simulink model "boost_inverter_control"  (R2018a)
settings: Solver=FixedStepAuto  StartTime=0.0  StopTime=0.5  FixedStep=1e-5  RelTol=1e-3  EnableMultiTasking=on
undefined symbols (not defined in the file): a, C, ki, kp, L, R, Wg
libraries: powerlib_meascontrol x4, simulink x1
settings Model: Creator=PC  LastModifiedBy=yassine
settings OptimizationCC: LifeSpan=inf
settings DebuggingCC: SFUnexpectedBacktrackingDiag=warning  SFNoUnconditionalDefaultTransitionDiag=warning
settings CodeAppCC: StateflowObjectComments=on
settings GRTTargetCC: TargetLangStandard=C89/C90 (ANSI)
settings ConfigComp: CovMetricSettings=dw  CovSaveCumulativeToWorkspaceVar=on  CovSaveSingleToWorkspaceVar=on  CovExternalEMLEnable=off

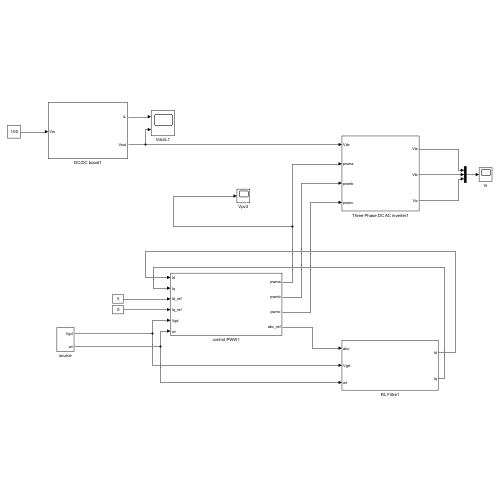
[thumbnail: Simulink's stored preview of the top-level diagram]
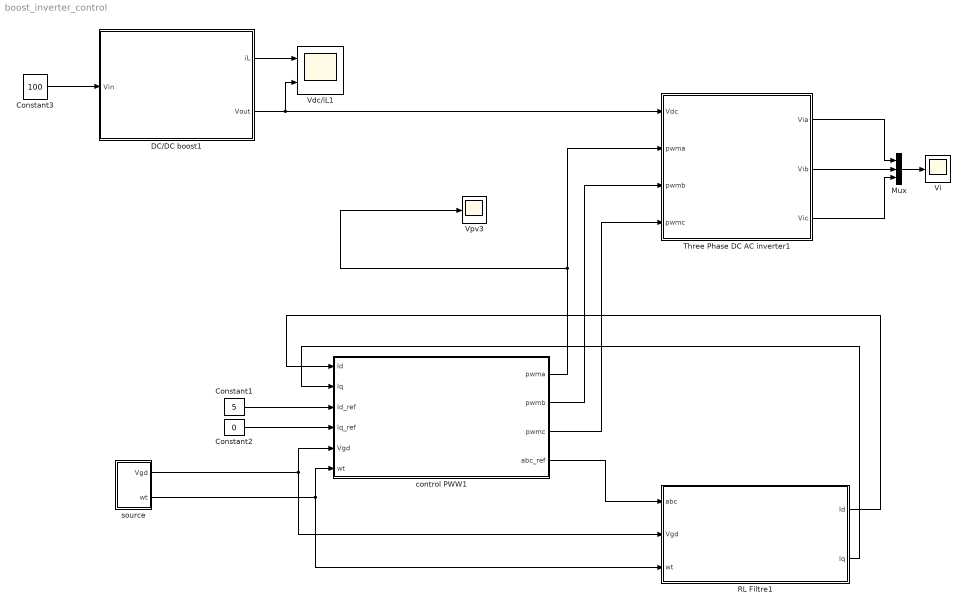
== system boost_inverter_control ==
  Constant1 : Constant  Value=5
  Constant2 : Constant  Value=0
  Constant3 : Constant  Value=100
  DC/DC boost1 : Subsystem  InitFcn=|
      | dv=0.5;
      | di=0.1;
      | F=20e3;
      | T=1/F;
      | Vs=230;
      | Vab=sqrt(3)*Vs;
      | Vdc=2*sqrt(2)*Vab/sqrt(3);
      | Vpv=100;
      | a=1-Vpv/Vdc;
      | Pn=200*5;
      | R=Vdc*Vdc/Pn;
      | L=0.5*Vpv*a*T/di;
      | C=0.5*Vdc*a*T/(dv*R);
  Mux : Mux  Inputs=3
  RL Filtre1 : Subsystem  InitFcn=|
      | fs=5000;
      | fe=50;
      | Wg=2*pi*fs;
      | Ig=2*Pn/(3*230*sqrt(2));
      | dIg=0.05*Ig;
      | L_=230*sqrt(3)/(6*sqrt(2)*fs*dIg);
      | r=0.01;
  Three Phase DC AC inverter1 : Subsystem
  Vdc/iL1 : Scope  NumInputPorts=2
  Vi : Scope
  Vpv3 : Scope
  control PWW1 : Subsystem  InitFcn=|
      | fs=5000;
      | fe=50;
      | Wg=2*pi*fe;
      | Ig=2*Pn/(3*230*sqrt(2));
      | dIg=0.05*Ig;
      | L=230*sqrt(3)/(6*sqrt(2)*fs*dIg);
      | Id_=5;
      | Iq_=0;
      | R=0.01;
      | tr=10e-5;
      | Te=tr/3;
      | ki=R/Te;
      | kp=L/Te;
  source : Subsystem
  wires:
  RL Filtre1/1(Id) -> control PWW1/1(Id)
  RL Filtre1/2(Iq) -> control PWW1/2(Iq)
  source/1(Vgd) -> control PWW1/5(Vgd), RL Filtre1/2(Vgd)
  Constant2/1 -> control PWW1/4(Iq_ref)
  Constant1/1 -> control PWW1/3(Id_ref)
  control PWW1/3(pwmc) -> Three Phase DC AC inverter1/4(pwmc)
  control PWW1/2(pwmb) -> Three Phase DC AC inverter1/3(pwmb)
  control PWW1/1(pwma) -> Three Phase DC AC inverter1/2(pwma), Vpv3/1
  DC/DC boost1/1(iL) -> Vdc/iL1/1
  Constant3/1 -> DC/DC boost1/1(Vin)
  Three Phase DC AC inverter1/1(Via) -> Mux/1
  Three Phase DC AC inverter1/2(Vib) -> Mux/2
  DC/DC boost1/2(Vout) -> Three Phase DC AC inverter1/1(Vdc), Vdc/iL1/2
  source/2(wt) -> control PWW1/6(wt), RL Filtre1/3(wt)
  control PWW1/4(abc_ref) -> RL Filtre1/1(abc)
  Mux/1 -> Vi/1
  Three Phase DC AC inverter1/3(Vic) -> Mux/3

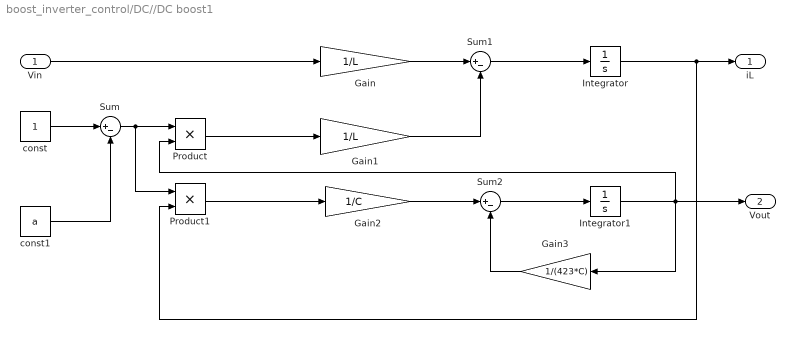
== system boost_inverter_control/DC//DC boost1 ==
  Vin : Inport
  Gain : Gain  Gain=1/L
  Gain1 : Gain  Gain=1/L
  Gain2 : Gain  Gain=1/C
  Gain3 : Gain  Gain=1/(423*C)
  Integrator : Integrator
  Integrator1 : Integrator
  Product : Product
  Product1 : Product
  Sum : Sum  Inputs=|+-
  Sum1 : Sum  Inputs=|+-
  Sum2 : Sum  Inputs=|+-
  const : Constant
  const1 : Constant  Value=a
  iL : Outport
  Vout : Outport  Port=2
  wires:
  Gain3/1 -> Sum2/2
  Integrator1/1 -> Vout/1, Product/2, Gain3/1
  Sum2/1 -> Integrator1/1
  Integrator/1 -> iL/1, Product1/2
  Vin/1 -> Gain/1
  const/1 -> Sum/1
  Product1/1 -> Gain2/1
  Product/1 -> Gain1/1
  Sum1/1 -> Integrator/1
  Gain1/1 -> Sum1/2
  Sum/1 -> Product/1, Product1/1
  Gain2/1 -> Sum2/1
  Gain/1 -> Sum1/1
  const1/1 -> Sum/2

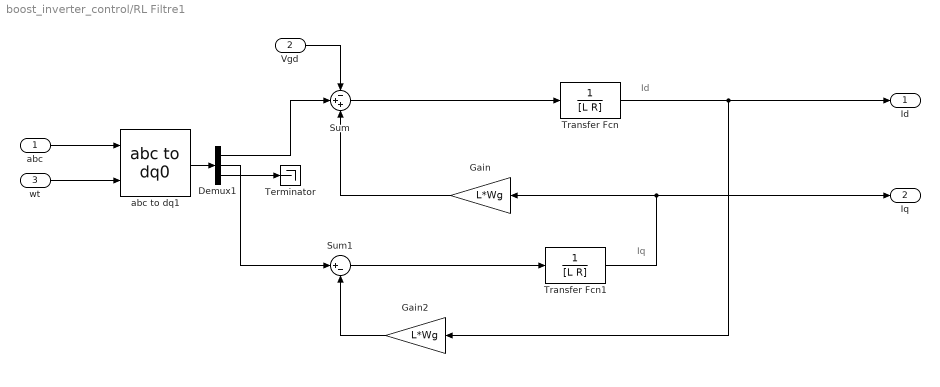
== system boost_inverter_control/RL Filtre1 ==
  note: Id
  note: Iq
  abc : Inport
  Vgd : Inport  Port=2
  wt : Inport  Port=3
  Demux1 : Demux  Outputs=3
  Gain : Gain  Gain=L*Wg
  Gain2 : Gain  Gain=L*Wg
  Sum : Sum  Inputs=-++
  Sum1 : Sum  Inputs=|+-
  Terminator : Terminator
  Transfer Fcn : TransferFcn  Denominator=[L R]
  Transfer Fcn1 : TransferFcn  Denominator=[L R]
  abc to dq1 : powerlib_meascontrol/Transformations/abc to dq0  Alignment=90 degrees behind phase A axis
  Id : Outport
  Iq : Outport  Port=2
  wires:
  Transfer Fcn/1 -> Gain2/1, Id/1
  Transfer Fcn1/1 -> Gain/1, Iq/1
  Demux1/1 -> Sum/2
  Demux1/2 -> Sum1/1
  abc to dq1/1 -> Demux1/1
  Demux1/3 -> Terminator/1
  abc/1 -> abc to dq1/1
  wt/1 -> abc to dq1/2
  Sum/1 -> Transfer Fcn/1
  Sum1/1 -> Transfer Fcn1/1
  Vgd/1 -> Sum/1
  Gain/1 -> Sum/3
  Gain2/1 -> Sum1/2

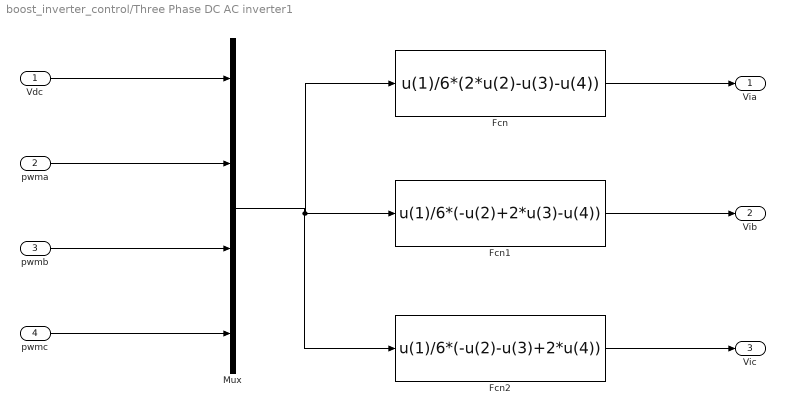
== system boost_inverter_control/Three Phase DC AC inverter1 ==
  Vdc : Inport
  pwma : Inport  Port=2
  pwmb : Inport  Port=3
  pwmc : Inport  Port=4
  Fcn : Fcn  Expr=u(1)/6*(2*u(2)-u(3)-u(4))
  Fcn1 : Fcn  Expr=u(1)/6*(-u(2)+2*u(3)-u(4))
  Fcn2 : Fcn  Expr=u(1)/6*(-u(2)-u(3)+2*u(4))
  Mux : Mux
  Via : Outport
  Vib : Outport  Port=2
  Vic : Outport  Port=3
  wires:
  Vdc/1 -> Mux/1
  Mux/1 -> Fcn2/1, Fcn1/1, Fcn/1
  Fcn2/1 -> Vic/1
  Fcn1/1 -> Vib/1
  Fcn/1 -> Via/1
  pwma/1 -> Mux/2
  pwmb/1 -> Mux/3
  pwmc/1 -> Mux/4

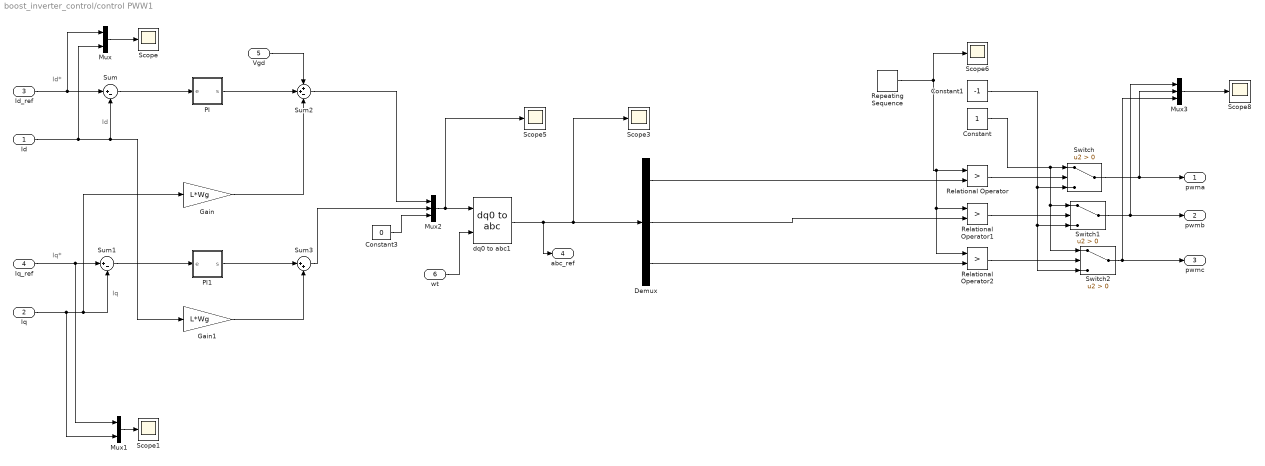
== system boost_inverter_control/control PWW1 ==
  note: Iq
  note: Iq*
  note: Id
  note: Id*
  Id : Inport
  Iq : Inport  Port=2
  Id_ref : Inport  Port=3
  Iq_ref : Inport  Port=4
  Vgd : Inport  Port=5
  wt : Inport  Port=6
  Constant : Constant
  Constant1 : Constant  Value=-1
  Constant3 : Constant  Value=0
  Demux : Demux  Outputs=3
  Gain : Gain  Gain=L*Wg
  Gain1 : Gain  Gain=L*Wg
  Mux : Mux  Inputs=2
  Mux1 : Mux  Inputs=2
  Mux2 : Mux  Inputs=3
  Mux3 : Mux  Inputs=3
  PI : Subsystem
  PI1 : Subsystem
  Relational Operator : RelationalOperator  Operator=>  OutDataTypeStr=boolean  RndMeth=Nearest
  Relational Operator1 : RelationalOperator  Operator=>  OutDataTypeStr=boolean  RndMeth=Nearest
  Relational Operator2 : RelationalOperator  Operator=>  OutDataTypeStr=boolean  RndMeth=Nearest
  Repeating Sequence : simulink/Sources/Repeating Sequence  rep_seq_t=[0 1/5000]  rep_seq_y=[1 -1]
  Scope{,1,3,5..6,8} (6 alike) : Scope
  Sum : Sum  Inputs=|+-
  Sum1 : Sum  Inputs=|+-
  Sum2 : Sum  Inputs=++-
  Sum3 : Sum  Inputs=|++
  Switch : Switch  Criteria=u2 > Threshold
  Switch1 : Switch  Criteria=u2 > Threshold
  Switch2 : Switch  Criteria=u2 > Threshold
  dq0 to abc1 : powerlib_meascontrol/Transformations/dq0 to abc  Alignment=90 degrees behind phase A axis
  pwma : Outport
  pwmb : Outport  Port=2
  pwmc : Outport  Port=3
  abc_ref : Outport  Port=4
  wires:
  Sum1/1 -> PI1/1(e)
  Id/1 -> Mux/2, Gain1/1, Sum/2
  Sum/1 -> PI/1(e)
  PI/1(s) -> Sum2/2
  Iq_ref/1 -> Mux1/1, Sum1/1
  Mux/1 -> Scope/1
  Iq/1 -> Mux1/2, Gain/1, Sum1/2
  Mux1/1 -> Scope1/1
  PI1/1(s) -> Sum3/1
  Constant3/1 -> Mux2/3
  Id_ref/1 -> Mux/1, Sum/1
  Repeating Sequence/1 -> Scope6/1, Relational Operator2/1, Relational Operator1/1, Relational Operator/1
  Demux/1 -> Relational Operator/2
  Demux/2 -> Relational Operator1/2
  Demux/3 -> Relational Operator2/2
  Switch2/1 -> Mux3/3, pwmc/1
  Switch1/1 -> Mux3/1, pwmb/1
  Switch/1 -> Mux3/2, pwma/1
  Relational Operator/1 -> Switch/2
  Constant/1 -> Switch1/1, Switch2/1, Switch/1
  Constant1/1 -> Switch/3, Switch1/3, Switch2/3
  Relational Operator1/1 -> Switch1/2
  Relational Operator2/1 -> Switch2/2
  Mux2/1 -> dq0 to abc1/1, Scope5/1
  Sum2/1 -> Mux2/1
  Sum3/1 -> Mux2/2
  Vgd/1 -> Sum2/1
  Gain/1 -> Sum2/3
  Gain1/1 -> Sum3/2
  dq0 to abc1/1 -> abc_ref/1, Scope3/1, Demux/1
  wt/1 -> dq0 to abc1/2
  Mux3/1 -> Scope8/1

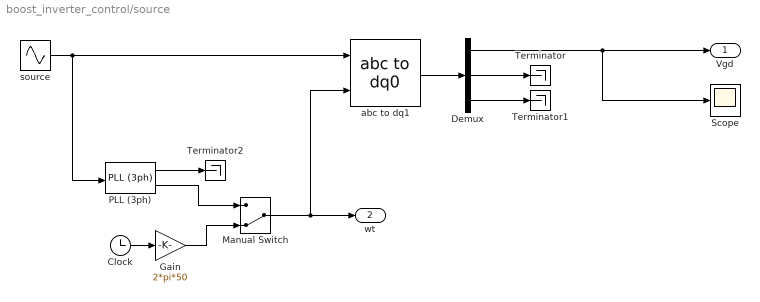
== system boost_inverter_control/source ==
  Clock : Clock
  Demux : Demux  Outputs=3
  Gain : Gain  Gain=2*pi*50
  Manual Switch : ManualSwitch  CurrentSetting=0
  PLL (3ph) : powerlib_meascontrol/PLL/PLL (3ph)  Fmin=45  Par_Init=[0, 50]  ParK=[180, 3200, 1]  TcD=1e-4  MaxRateChangeFreq=12  FilterCutOffFreq=25  Ts=0  AGC=on
  Scope : Scope
  Terminator : Terminator
  Terminator1 : Terminator
  Terminator2 : Terminator
  abc to dq1 : powerlib_meascontrol/Transformations/abc to dq0  Alignment=90 degrees behind phase A axis
  source : Sin  Amplitude=230*sqrt(2)  Frequency=2*pi*50  Phase=[0 -2*pi/3 2*pi/3]  SampleTime=0
  Vgd : Outport
  wt : Outport  Port=2
  wires:
  abc to dq1/1 -> Demux/1
  source/1 -> abc to dq1/1, PLL (3ph)/1
  Demux/2 -> Terminator/1
  Demux/3 -> Terminator1/1
  Demux/1 -> Scope/1, Vgd/1
  PLL (3ph)/1 -> Terminator2/1
  Clock/1 -> Gain/1
  PLL (3ph)/2 -> Manual Switch/1
  Gain/1 -> Manual Switch/2
  Manual Switch/1 -> wt/1, abc to dq1/2

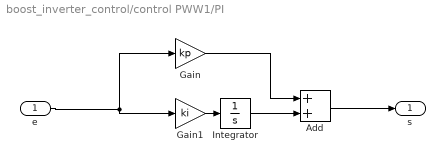
== system boost_inverter_control/control PWW1/PI ==
  e : Inport
  Add : Sum
  Gain : Gain  Gain=kp
  Gain1 : Gain  Gain=ki
  Integrator : Integrator  UpperSaturationLimit=350  LowerSaturationLimit=-350
  s : Outport
  wires:
  Gain/1 -> Add/1
  Gain1/1 -> Integrator/1
  Integrator/1 -> Add/2
  e/1 -> Gain/1, Gain1/1
  Add/1 -> s/1

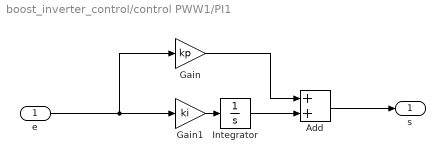
== system boost_inverter_control/control PWW1/PI1 ==
  e : Inport
  Add : Sum
  Gain : Gain  Gain=kp
  Gain1 : Gain  Gain=ki
  Integrator : Integrator  UpperSaturationLimit=350  LowerSaturationLimit=-350
  s : Outport
  wires:
  Add/1 -> s/1
  e/1 -> Gain/1, Gain1/1
  Integrator/1 -> Add/2
  Gain1/1 -> Integrator/1
  Gain/1 -> Add/1
